simulink model "invertedPendolum"  (R2019b)
settings: Solver=VariableStepAuto  StartTime=0.0  StopTime=60  FixedStep=0.0001  RelTol=1e-4
InitFcn:
  | simulationVar
values from neighbouring files (symbols this model uses):
  tauMotMax = Ka * Id    (= 6208417600)    [simulationVar.m]
undefined symbols (not defined in the file or in its folder): smiData, X, Y, Z
libraries: sm_lib x768, simulink x6, nesl_utility x3
(part 1 of 13)
settings Model: Creator=alfyhack  LastModifiedBy=socci
settings SolverCC: AlgebraicLoopSolver=LineSearch
settings DebuggingCC: UnderSpecifiedDimensionMsg=warning
settings SFSimCC: CustomCodeUndefinedFunction=UseInterfaceOnly

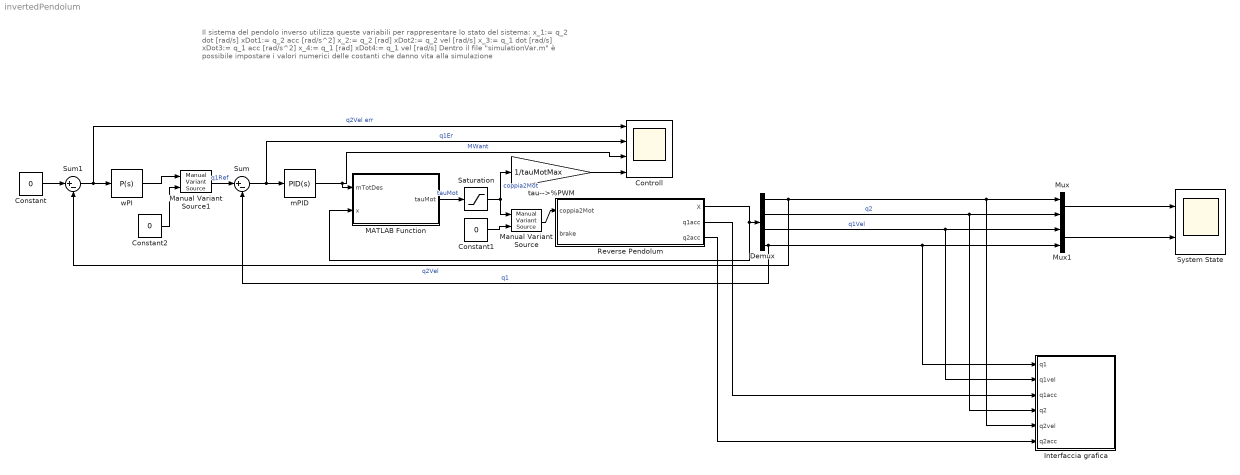
== system invertedPendolum ==
  note: Il sistema del pendolo inverso utilizza queste variabili per rappresentare lo stato del sistema:
      |
      | x_1:= q_2 dot  [rad/s]		xDot1:= q_2 acc   [rad/s^2]
      | x_2:= q_2        [rad]		xDot2:= q_2 vel    [rad/s]
      | x_3:= q_1 dot  [rad/s]		xDot3:= q_1 acc   [rad/s^2]
      | x_4:= q_1        [rad]		xDot4:= q_1 vel    [rad/s]
      |
      | Dentro il file "simulationVar.m" è possibile impostare i valori numerici delle costanti che danno vita alla simulazione
  Constant : Constant  Value=0
  Constant1 : Constant  Value=0
  Constant2 : Constant  Value=0
  Controll : Scope  NumInputPorts=4
  Demux : Demux
  Interfaccia grafica : Subsystem
  MATLAB Function : MATLAB Function  TreatAsAtomicUnit=on
  Manual Variant Source : simulink/Signal Routing/Manual Variant Source  NumChoices=2  LabelModeActiveChoice=V_1
      settings: SourceProductName=Simulink
  Manual Variant Source1 : simulink/Signal Routing/Manual Variant Source  NumChoices=2  LabelModeActiveChoice=V_1
      settings: SourceProductName=Simulink
  Mux : Mux  Inputs=2
  Mux1 : Mux  Inputs=2
  Reverse Pendolum : Subsystem
  Saturation : Saturate  UpperLimit=tauMotMax  LowerLimit=-tauMotMax
  Sum : Sum  Inputs=|+-
  Sum1 : Sum  Inputs=|+-
  System State : Scope  NumInputPorts=2
  mPID : simulink/Continuous/PID Controller  Controller=PID  Form=Parallel  TimeDomain=Continuous-time  SampleTime=-1  IntegratorMethod=Forward Euler  FilterMethod=Forward Euler  ControllerParametersSource=internal  P=44059890.2523914  I=6444277.98639226  D=74154463.3015082  UseFilter=on  N=34.9657186034109  TunerSelectOption=Transfer Function Based (PID Tuner App)  InitialConditionSource=internal  InitialConditionForIntegrator=0  InitialConditionForFilter=0  DifferentiatorICPrevScaledInput=0  ExternalReset=none  TrackingMode=off  Kt=1  LimitOutput=off  UpperSaturationLimit=1000  LowerSaturationLimit=1000  LinearizeAsGain=off  AntiWindupMode=none  Kb=1  POutMin=[]  POutMax=[]  IOutMin=[]  IOutMax=[]  DOutMin=[]  DOutMax=[]  NOutMin=[]  NOutMax=[]  SumOutMin=[]  SumOutMax=[]  SaturationOutMin=[]  SaturationOutMax=[]  PParamMin=[]  PParamMax=[]  IParamMin=[]  IParamMax=[]  DParamMin=[]  DParamMax=[]  NParamMin=[]  NParamMax=[]  KbParamMin=[]  KbParamMax=[]  KtParamMin=[]  KtParamMax=[]  KbOutMin=[]  KbOutMax=[]  KtOutMin=[]  KtOutMax=[]  IntegratorOutMin=[]  IntegratorOutMax=[]  FilterOutMin=[]  FilterOutMax=[]  SumI1OutMin=[]  SumI1OutMax=[]  SumI2OutMin=[]  SumI2OutMax=[]  SumI3OutMin=[]  SumI3OutMax=[]  SumI4OutMin=[]  SumI4OutMax=[]  SumDOutMin=[]  SumDOutMax=[]  DifferentiatorOutMin=[]  DifferentiatorOutMax=[]  FilterDiffOutCoefMin=[]  FilterDiffOutCoefMax=[]  ReciprocalOutMin=[]  ReciprocalOutMax=[]  SumDenOutMin=[]  SumDenOutMax=[]  SumNumOutMin=[]  SumNumOutMax=[]  DivideOutMin=[]  DivideOutMax=[]  IntegratorContinuousStateAttributes=''  IntegratorStateMustResolveToSignalObject=off  IntegratorRTWStateStorageClass=Auto  FilterContinuousStateAttributes=''  FilterStateMustResolveToSignalObject=off  FilterRTWStateStorageClass=Auto  ParallelPVariant=InternalParameters  IdealPVariant=Disabled  IVariant=InternalParameters  DVariant=InternalParameters  IntegratorVariant=Continuous  SatVariant=Disabled  AWVariant=Passthrough  PCopyVariant=Disabled  TRVariant=Disabled  FdbkBlocksVariant=Forward  IdealPFdbkVariant=Disabled  SatFdbkVariant=Disabled  DerivativeFilterVariant=ContFilter  NVariant=InternalParameters  NCopyVariant=Disabled  FilterICVariant=InternalICsFilter  IntegratorICVariant=InternalICs  ExternalResetVariant=Disabled  TRSumVariant=Passthrough  SumFdbkVariant=Disabled  SumVariant=Sum_PID
  tau-->%PWM : Gain  Gain=1/tauMotMax
  wPI : simulink/Continuous/PID Controller  Controller=P  Form=Parallel  TimeDomain=Continuous-time  SampleTime=-1  IntegratorMethod=Forward Euler  FilterMethod=Forward Euler  ControllerParametersSource=internal  P=0.000273498312206375  I=0.001  D=1  UseFilter=on  N=2000  TunerSelectOption=Transfer Function Based (PID Tuner App)  InitialConditionSource=internal  InitialConditionForIntegrator=0  InitialConditionForFilter=0  DifferentiatorICPrevScaledInput=0  ExternalReset=none  TrackingMode=off  Kt=1  LimitOutput=on  UpperSaturationLimit=0.1  LowerSaturationLimit=-0.1  LinearizeAsGain=off  AntiWindupMode=none  Kb=1  POutMin=[]  POutMax=[]  IOutMin=[]  IOutMax=[]  DOutMin=[]  DOutMax=[]  NOutMin=[]  NOutMax=[]  SumOutMin=[]  SumOutMax=[]  SaturationOutMin=[]  SaturationOutMax=[]  PParamMin=[]  PParamMax=[]  IParamMin=[]  IParamMax=[]  DParamMin=[]  DParamMax=[]  NParamMin=[]  NParamMax=[]  KbParamMin=[]  KbParamMax=[]  KtParamMin=[]  KtParamMax=[]  KbOutMin=[]  KbOutMax=[]  KtOutMin=[]  KtOutMax=[]  IntegratorOutMin=[]  IntegratorOutMax=[]  FilterOutMin=[]  FilterOutMax=[]  SumI1OutMin=[]  SumI1OutMax=[]  SumI2OutMin=[]  SumI2OutMax=[]  SumI3OutMin=[]  SumI3OutMax=[]  SumI4OutMin=[]  SumI4OutMax=[]  SumDOutMin=[]  SumDOutMax=[]  DifferentiatorOutMin=[]  DifferentiatorOutMax=[]  FilterDiffOutCoefMin=[]  FilterDiffOutCoefMax=[]  ReciprocalOutMin=[]  ReciprocalOutMax=[]  SumDenOutMin=[]  SumDenOutMax=[]  SumNumOutMin=[]  SumNumOutMax=[]  DivideOutMin=[]  DivideOutMax=[]  IntegratorContinuousStateAttributes=''  IntegratorStateMustResolveToSignalObject=off  IntegratorRTWStateStorageClass=Auto  FilterContinuousStateAttributes=''  FilterStateMustResolveToSignalObject=off  FilterRTWStateStorageClass=Auto  ParallelPVariant=InternalParameters  IdealPVariant=Disabled  IVariant=Disabled  DVariant=Disabled  IntegratorVariant=Disabled  SatVariant=Enabled  AWVariant=Disabled  PCopyVariant=Disabled  TRVariant=Disabled  FdbkBlocksVariant=Forward  IdealPFdbkVariant=Disabled  SatFdbkVariant=Disabled  DerivativeFilterVariant=Disabled  NVariant=Disabled  NCopyVariant=Disabled_SignalSpec  FilterICVariant=Disabled  IntegratorICVariant=Disabled  ExternalResetVariant=Disabled  TRSumVariant=Passthrough  SumFdbkVariant=Disabled  SumVariant=Passthrough_P
  wires:
  Demux/4 -> Interfaccia grafica/1(q1), Mux1/2, Sum/2  "q1"
  Demux/1 -> Interfaccia grafica/5(q2vel), Mux/1, Sum1/2  "q2Vel"
  MATLAB Function/1(tauMot) -> Saturation/1  "tauMot"
  mPID/1 -> Controll/3, MATLAB Function/1(mTotDes)  "MWant"
  Sum/1 -> Controll/2, mPID/1  "q1Er"
  wPI/1 -> Manual Variant Source1/1
  Constant/1 -> Sum1/1
  Sum1/1 -> Controll/1, wPI/1  "q2Vel err"
  Saturation/1 -> tau-->%PWM/1, Manual Variant Source/1  "coppia2Mot"
  Reverse Pendolum/1(X) -> Demux/1, MATLAB Function/2(x)
  Demux/3 -> Interfaccia grafica/2(q1vel), Mux1/1  "q1Vel"
  Mux1/1 -> System State/2
  Mux/1 -> System State/1
  tau-->%PWM/1 -> Controll/4
  Manual Variant Source/1 -> Reverse Pendolum/1(coppia2Mot)
  Constant1/1 -> Manual Variant Source/2
  Manual Variant Source1/1 -> Sum/1  "q1Ref"
  Constant2/1 -> Manual Variant Source1/2
  Demux/2 -> Interfaccia grafica/4(q2), Mux/2  "q2"
  Reverse Pendolum/2(q1acc) -> Interfaccia grafica/3(q1acc)
  Reverse Pendolum/3(q2acc) -> Interfaccia grafica/6(q2acc)

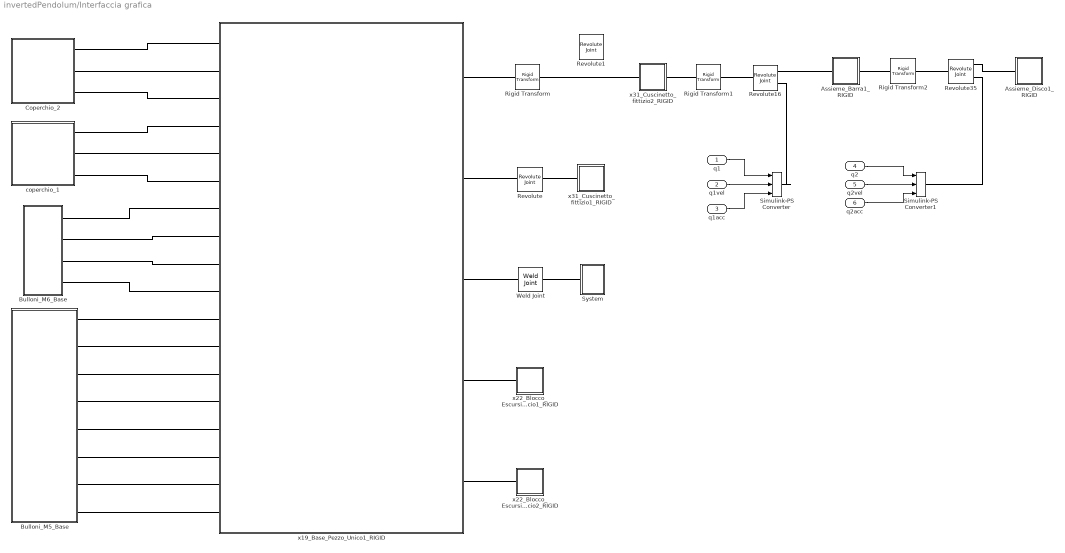
== system invertedPendolum/Interfaccia grafica ==
  q1 : Inport
  q1vel : Inport  Port=2
  q1acc : Inport  Port=3
  q2 : Inport  Port=4
  q2vel : Inport  Port=5
  q2acc : Inport  Port=6
  Assieme_Barra1_RIGID : Subsystem
  Assieme_Disco1_RIGID : Subsystem
  Bulloni_M5_Base : Subsystem
  Bulloni_M6_Base : Subsystem
  Coperchio_2 : Subsystem
  Revolute : sm_lib/Joints/Revolute Joint  JointMode=Normal  SenseConstraintForce=off  SenseConstraintForceX=off  SenseConstraintForceY=off  SenseConstraintForceZ=off  SenseConstraintTorque=off  SenseConstraintTorqueX=off  SenseConstraintTorqueY=off  SenseConstraintTorqueZ=off  SenseTotalForce=off  SenseTotalForceX=off  SenseTotalForceY=off  SenseTotalForceZ=off  SenseTotalTorque=off  SenseTotalTorqueX=off  SenseTotalTorqueY=off  SenseTotalTorqueZ=off  CompositeWrenchDir=FollowerOnBase  CompositeWrenchFrame=BaseFrame  EquilibriumPosition=0  EquilibriumPositionUnits=rad  SpringStiffness=0  SpringStiffnessUnits=N*m/rad  DampingCoefficient=0  DampingCoefficientUnits=N*m/(rad/s)  TorqueActuationMode=NoTorque  MotionActuationMode=ComputedMotion  SensePosition=off  SenseVelocity=off  SenseAcceleration=off  SenseTorqueForce=off  SenseLowerLimitTorqueForce=off  SenseUpperLimitTorqueForce=off  LowerLimitSpecify=off  LowerLimitBound=-90  LowerLimitBoundUnits=deg  LowerLimitStiffness=1e4  LowerLimitStiffnessUnits=N*m/deg  LowerLimitDamping=10  LowerLimitDampingUnits=N*m/(deg/s)  LowerLimitTransitionRegionWidth=0.1  LowerLimitTransitionRegionWidthUnits=deg  UpperLimitSpecify=off  UpperLimitBound=90  UpperLimitBoundUnits=deg  UpperLimitStiffness=1e4  UpperLimitStiffnessUnits=N*m/deg  UpperLimitDamping=10  UpperLimitDampingUnits=N*m/(deg/s)  UpperLimitTransitionRegionWidth=0.1  UpperLimitTransitionRegionWidthUnits=deg  PositionTargetSpecify=on  PositionTargetPriority=Low  PositionTargetValue=smiData.RevoluteJoint(1).Rz.Pos  PositionTargetValueUnits=deg  VelocityTargetSpecify=off  VelocityTargetPriority=High  VelocityTargetValue=0  VelocityTargetValueUnits=deg/s
  Revolute1 : sm_lib/Joints/Revolute Joint  JointMode=Normal  SenseConstraintForce=off  SenseConstraintForceX=off  SenseConstraintForceY=off  SenseConstraintForceZ=off  SenseConstraintTorque=off  SenseConstraintTorqueX=off  SenseConstraintTorqueY=off  SenseConstraintTorqueZ=off  SenseTotalForce=off  SenseTotalForceX=off  SenseTotalForceY=off  SenseTotalForceZ=off  SenseTotalTorque=off  SenseTotalTorqueX=off  SenseTotalTorqueY=off  SenseTotalTorqueZ=off  CompositeWrenchDir=FollowerOnBase  CompositeWrenchFrame=BaseFrame  EquilibriumPosition=0  EquilibriumPositionUnits=rad  SpringStiffness=0  SpringStiffnessUnits=N*m/rad  DampingCoefficient=0  DampingCoefficientUnits=N*m/(rad/s)  TorqueActuationMode=NoTorque  MotionActuationMode=ComputedMotion  SensePosition=off  SenseVelocity=off  SenseAcceleration=off  SenseTorqueForce=off  SenseLowerLimitTorqueForce=off  SenseUpperLimitTorqueForce=off  LowerLimitSpecify=off  LowerLimitBound=-90  LowerLimitBoundUnits=deg  LowerLimitStiffness=1e4  LowerLimitStiffnessUnits=N*m/deg  LowerLimitDamping=10  LowerLimitDampingUnits=N*m/(deg/s)  LowerLimitTransitionRegionWidth=0.1  LowerLimitTransitionRegionWidthUnits=deg  UpperLimitSpecify=off  UpperLimitBound=90  UpperLimitBoundUnits=deg  UpperLimitStiffness=1e4  UpperLimitStiffnessUnits=N*m/deg  UpperLimitDamping=10  UpperLimitDampingUnits=N*m/(deg/s)  UpperLimitTransitionRegionWidth=0.1  UpperLimitTransitionRegionWidthUnits=deg  PositionTargetSpecify=on  PositionTargetPriority=Low  PositionTargetValue=smiData.RevoluteJoint(2).Rz.Pos  PositionTargetValueUnits=deg  VelocityTargetSpecify=off  VelocityTargetPriority=High  VelocityTargetValue=0  VelocityTargetValueUnits=deg/s
  Revolute16 : sm_lib/Joints/Revolute Joint  JointMode=Normal  SenseConstraintForce=off  SenseConstraintForceX=off  SenseConstraintForceY=off  SenseConstraintForceZ=off  SenseConstraintTorque=off  SenseConstraintTorqueX=off  SenseConstraintTorqueY=off  SenseConstraintTorqueZ=off  SenseTotalForce=off  SenseTotalForceX=off  SenseTotalForceY=off  SenseTotalForceZ=off  SenseTotalTorque=off  SenseTotalTorqueX=off  SenseTotalTorqueY=off  SenseTotalTorqueZ=off  CompositeWrenchDir=FollowerOnBase  CompositeWrenchFrame=BaseFrame  EquilibriumPosition=0  EquilibriumPositionUnits=rad  SpringStiffness=0  SpringStiffnessUnits=N*m/rad  DampingCoefficient=0  DampingCoefficientUnits=N*m/(rad/s)  TorqueActuationMode=ComputedTorque  MotionActuationMode=InputMotion  SensePosition=off  SenseVelocity=off  SenseAcceleration=off  SenseTorqueForce=off  SenseLowerLimitTorqueForce=off  SenseUpperLimitTorqueForce=off  LowerLimitSpecify=off  LowerLimitBound=-90  LowerLimitBoundUnits=deg  LowerLimitStiffness=1e4  LowerLimitStiffnessUnits=N*m/deg  LowerLimitDamping=10  LowerLimitDampingUnits=N*m/(deg/s)  LowerLimitTransitionRegionWidth=0.1  LowerLimitTransitionRegionWidthUnits=deg  UpperLimitSpecify=off  UpperLimitBound=90  UpperLimitBoundUnits=deg  UpperLimitStiffness=1e4  UpperLimitStiffnessUnits=N*m/deg  UpperLimitDamping=10  UpperLimitDampingUnits=N*m/(deg/s)  UpperLimitTransitionRegionWidth=0.1  UpperLimitTransitionRegionWidthUnits=deg  PositionTargetSpecify=on  PositionTargetPriority=Low  PositionTargetValue=smiData.RevoluteJoint(17).Rz.Pos  PositionTargetValueUnits=deg  VelocityTargetSpecify=off  VelocityTargetPriority=High  VelocityTargetValue=0  VelocityTargetValueUnits=deg/s
  Revolute35 : sm_lib/Joints/Revolute Joint  JointMode=Normal  SenseConstraintForce=off  SenseConstraintForceX=off  SenseConstraintForceY=off  SenseConstraintForceZ=off  SenseConstraintTorque=off  SenseConstraintTorqueX=off  SenseConstraintTorqueY=off  SenseConstraintTorqueZ=off  SenseTotalForce=off  SenseTotalForceX=off  SenseTotalForceY=off  SenseTotalForceZ=off  SenseTotalTorque=off  SenseTotalTorqueX=off  SenseTotalTorqueY=off  SenseTotalTorqueZ=off  CompositeWrenchDir=FollowerOnBase  CompositeWrenchFrame=BaseFrame  EquilibriumPosition=0  EquilibriumPositionUnits=rad  SpringStiffness=0  SpringStiffnessUnits=N*m/rad  DampingCoefficient=0  DampingCoefficientUnits=N*m/(rad/s)  TorqueActuationMode=ComputedTorque  MotionActuationMode=InputMotion  SensePosition=off  SenseVelocity=off  SenseAcceleration=off  SenseTorqueForce=off  SenseLowerLimitTorqueForce=off  SenseUpperLimitTorqueForce=off  LowerLimitSpecify=off  LowerLimitBound=-90  LowerLimitBoundUnits=deg  LowerLimitStiffness=1e4  LowerLimitStiffnessUnits=N*m/deg  LowerLimitDamping=10  LowerLimitDampingUnits=N*m/(deg/s)  LowerLimitTransitionRegionWidth=0.1  LowerLimitTransitionRegionWidthUnits=deg  UpperLimitSpecify=off  UpperLimitBound=90  UpperLimitBoundUnits=deg  UpperLimitStiffness=1e4  UpperLimitStiffnessUnits=N*m/deg  UpperLimitDamping=10  UpperLimitDampingUnits=N*m/(deg/s)  UpperLimitTransitionRegionWidth=0.1  UpperLimitTransitionRegionWidthUnits=deg  PositionTargetSpecify=on  PositionTargetPriority=Low  PositionTargetValue=smiData.RevoluteJoint(36).Rz.Pos  PositionTargetValueUnits=deg  VelocityTargetSpecify=off  VelocityTargetPriority=High  VelocityTargetValue=0  VelocityTargetValueUnits=deg/s
  Rigid Transform : sm_lib/Frames and Transforms/Rigid Transform  TranslationMethod=None  TranslationStandardOffset=0  TranslationLengthUnit=m  TranslationStandardAxis=+Z  TranslationCartesianOffset=[0 0 0]  TranslationROffset=0  TranslationROffsetUnits=m  TranslationZOffset=0  TranslationZOffsetUnits=m  TranslationThetaOffset=0  TranslationThetaOffsetUnits=deg  RotationMethod=None  RotationAngleUnits=deg  RotationStandardAxis=+Z  RotationAngle=0.0  RotationArbitraryAxis=[0 0 1]  FollAlignAxisA=+X  BaseAlignAxisA=+Y  FollAlignAxisB=+Y  BaseAlignAxisB=+Z  RotationSequenceAxes=FollowerAxes  RotationSequence=XYX  RotationSequenceAngles=[0 0 0]  RotationSequenceAnglesUnits=deg  RotationMatrix=[1 0 0; 0 1 0; 0 0 1]
  Rigid Transform1 : sm_lib/Frames and Transforms/Rigid Transform  TranslationMethod=None  TranslationStandardOffset=0  TranslationLengthUnit=m  TranslationStandardAxis=+Z  TranslationCartesianOffset=[0 0 0]  TranslationROffset=0  TranslationROffsetUnits=m  TranslationZOffset=0  TranslationZOffsetUnits=m  TranslationThetaOffset=0  TranslationThetaOffsetUnits=deg  RotationMethod=None  RotationAngleUnits=deg  RotationStandardAxis=+Z  RotationAngle=0.0  RotationArbitraryAxis=[0 0 1]  FollAlignAxisA=+X  BaseAlignAxisA=+Y  FollAlignAxisB=+Y  BaseAlignAxisB=+Z  RotationSequenceAxes=FollowerAxes  RotationSequence=XYX  RotationSequenceAngles=[0 0 0]  RotationSequenceAnglesUnits=deg  RotationMatrix=[1 0 0; 0 1 0; 0 0 1]
  Rigid Transform2 : sm_lib/Frames and Transforms/Rigid Transform  TranslationMethod=None  TranslationStandardOffset=0  TranslationLengthUnit=m  TranslationStandardAxis=+Z  TranslationCartesianOffset=[0 0 0]  TranslationROffset=0  TranslationROffsetUnits=m  TranslationZOffset=0  TranslationZOffsetUnits=m  TranslationThetaOffset=0  TranslationThetaOffsetUnits=deg  RotationMethod=None  RotationAngleUnits=deg  RotationStandardAxis=+Z  RotationAngle=0.0  RotationArbitraryAxis=[0 0 1]  FollAlignAxisA=+X  BaseAlignAxisA=+Y  FollAlignAxisB=+Y  BaseAlignAxisB=+Z  RotationSequenceAxes=FollowerAxes  RotationSequence=XYX  RotationSequenceAngles=[0 0 0]  RotationSequenceAnglesUnits=deg  RotationMatrix=[1 0 0; 0 1 0; 0 0 1]
  Simulink-PS Converter : nesl_utility/Simulink-PS Converter  PhysicalDomain=network_engine_domain  SubClassName=ps_input  LeftPortType=input  RightPortType=output  PseudoPeriodic=off  Frequencies=[]  NoiseDistribution=none  NoiseParameters=[]  Unit=1  AffineConversion=off  FilteringAndDerivatives=provide  SimscapeFilterOrder=1  InputFilterTimeConstant=0.001  UdotUserProvided=2
  Simulink-PS Converter1 : nesl_utility/Simulink-PS Converter  PhysicalDomain=network_engine_domain  SubClassName=ps_input  LeftPortType=input  RightPortType=output  PseudoPeriodic=off  Frequencies=[]  NoiseDistribution=none  NoiseParameters=[]  Unit=1  AffineConversion=off  FilteringAndDerivatives=provide  SimscapeFilterOrder=1  InputFilterTimeConstant=0.001  UdotUserProvided=2
  System : Subsystem
  Weld Joint : sm_lib/Joints/Weld Joint  JointMode=Normal  SenseConstraintForce=off  SenseConstraintForceX=off  SenseConstraintForceY=off  SenseConstraintForceZ=off  SenseConstraintTorque=off  SenseConstraintTorqueX=off  SenseConstraintTorqueY=off  SenseConstraintTorqueZ=off  SenseTotalForce=off  SenseTotalForceX=off  SenseTotalForceY=off  SenseTotalForceZ=off  SenseTotalTorque=off  SenseTotalTorqueX=off  SenseTotalTorqueY=off  SenseTotalTorqueZ=off  CompositeWrenchDir=FollowerOnBase  CompositeWrenchFrame=BaseFrame
  coperchio_1 : Subsystem
  x19_Base_Pezzo_Unico1_RIGID : Subsystem
  x22_Blocco_Escursione_Braccio1_RIGID : Subsystem
  x22_Blocco_Escursione_Braccio2_RIGID : Subsystem
  x31_Cuscinetto_fittizio1_RIGID : Subsystem
  x31_Cuscinetto_fittizio2_RIGID : Subsystem
  wires:
  q1/1 -> Simulink-PS Converter/1
  q1vel/1 -> Simulink-PS Converter/2
  q1acc/1 -> Simulink-PS Converter/3
  q2/1 -> Simulink-PS Converter1/1
  q2vel/1 -> Simulink-PS Converter1/2
  q2acc/1 -> Simulink-PS Converter1/3
  connections:
  Bulloni_M5_Base/RConn4 -- x19_Base_Pezzo_Unico1_RIGID/LConn14
  Bulloni_M5_Base/RConn2 -- x19_Base_Pezzo_Unico1_RIGID/LConn12
  Bulloni_M6_Base/RConn1 -- x19_Base_Pezzo_Unico1_RIGID/LConn7
  coperchio_1/LConn1 -- x19_Base_Pezzo_Unico1_RIGID/LConn4
  Bulloni_M5_Base/RConn1 -- x19_Base_Pezzo_Unico1_RIGID/LConn11
  Coperchio_2/RConn2 -- x19_Base_Pezzo_Unico1_RIGID/LConn2
  Bulloni_M5_Base/RConn5 -- x19_Base_Pezzo_Unico1_RIGID/LConn15
  Bulloni_M5_Base/RConn6 -- x19_Base_Pezzo_Unico1_RIGID/LConn16
  Bulloni_M5_Base/RConn7 -- x19_Base_Pezzo_Unico1_RIGID/LConn17
  x22_Blocco_Escursione_Braccio1_RIGID/LConn1 -- x19_Base_Pezzo_Unico1_RIGID/RConn4
  Revolute/RConn1 -- x19_Base_Pezzo_Unico1_RIGID/RConn2
  coperchio_1/LConn3 -- x19_Base_Pezzo_Unico1_RIGID/LConn6
  Bulloni_M6_Base/RConn2 -- x19_Base_Pezzo_Unico1_RIGID/LConn8
  Weld Joint/LConn1 -- x19_Base_Pezzo_Unico1_RIGID/RConn3
  Bulloni_M5_Base/RConn3 -- x19_Base_Pezzo_Unico1_RIGID/LConn13
  Assieme_Disco1_RIGID/RConn1 -- Revolute35/LConn1
  Bulloni_M6_Base/RConn3 -- x19_Base_Pezzo_Unico1_RIGID/LConn9
  x19_Base_Pezzo_Unico1_RIGID/LConn18 -- Bulloni_M5_Base/RConn8
  coperchio_1/LConn2 -- x19_Base_Pezzo_Unico1_RIGID/LConn5
  Assieme_Barra1_RIGID/RConn1 -- Revolute16/LConn1
  x22_Blocco_Escursione_Braccio2_RIGID/LConn1 -- x19_Base_Pezzo_Unico1_RIGID/RConn5
  Bulloni_M6_Base/RConn4 -- x19_Base_Pezzo_Unico1_RIGID/LConn10
  Rigid Transform/LConn1 -- x19_Base_Pezzo_Unico1_RIGID/RConn1
  Revolute/LConn1 -- x31_Cuscinetto_fittizio1_RIGID/RConn1
  Coperchio_2/RConn1 -- x19_Base_Pezzo_Unico1_RIGID/LConn1
  Assieme_Barra1_RIGID/LConn1 -- Rigid Transform2/LConn1
  System/RConn1 -- Weld Joint/RConn1
  Rigid Transform1/LConn1 -- x31_Cuscinetto_fittizio2_RIGID/LConn1
  x19_Base_Pezzo_Unico1_RIGID/LConn3 -- Coperchio_2/RConn3
  Revolute16/RConn1 -- Rigid Transform1/RConn1
  Simulink-PS Converter/RConn1 -- Revolute16/LConn2
  Rigid Transform/RConn1 -- x31_Cuscinetto_fittizio2_RIGID/RConn1
  Simulink-PS Converter1/RConn1 -- Revolute35/LConn2
  Rigid Transform2/RConn1 -- Revolute35/RConn1

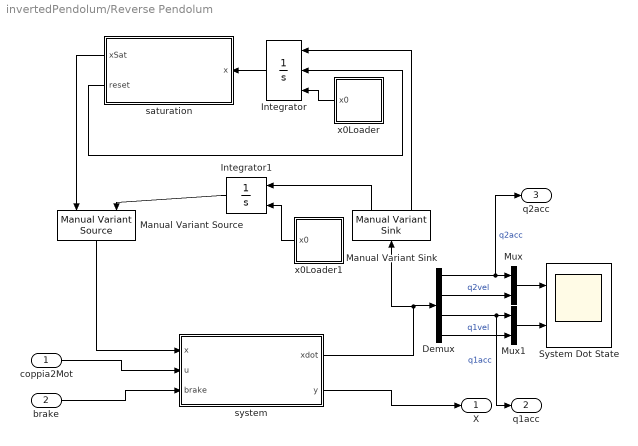
== system invertedPendolum/Reverse Pendolum ==
  coppia2Mot : Inport
  brake : Inport  Port=2
  Demux : Demux
  Integrator : Integrator  ExternalReset=rising  InitialConditionSource=external  InitialCondition=[0,0.1,0]
  Integrator1 : Integrator  InitialConditionSource=external
  Manual Variant Sink : simulink/Signal Routing/Manual Variant Sink  NumChoices=2  LabelModeActiveChoice=V_2
      settings: SourceProductName=Simulink
  Manual Variant Source : simulink/Signal Routing/Manual Variant Source  NumChoices=2  LabelModeActiveChoice=V_1
      settings: SourceProductName=Simulink
  Mux : Mux  Inputs=2
  Mux1 : Mux  Inputs=2
  System Dot State : Scope  NumInputPorts=2
  saturation : MATLAB Function  TreatAsAtomicUnit=on
  system : MATLAB Function  TreatAsAtomicUnit=on
  x0Loader : MATLAB Function  TreatAsAtomicUnit=on
  x0Loader1 : MATLAB Function  TreatAsAtomicUnit=on
  X : Outport  VectorParamsAs1DForOutWhenUnconnected=off
  q1acc : Outport  Port=2  VectorParamsAs1DForOutWhenUnconnected=off
  q2acc : Outport  Port=3  VectorParamsAs1DForOutWhenUnconnected=off
  wires:
  x0Loader/1(x0) -> Integrator/3
  Integrator/1 -> saturation/1(x)
  saturation/2(reset) -> Integrator/2
  coppia2Mot/1 -> system/2(u)
  system/2(y) -> X/1
  Mux/1 -> System Dot State/1
  Demux/3 -> q1acc/1, Mux1/1  "q1acc"
  Demux/1 -> q2acc/1, Mux/1  "q2acc"
  system/1(xdot) -> Manual Variant Sink/1, Demux/1
  Demux/2 -> Mux/2  "q2vel"
  Demux/4 -> Mux1/2  "q1vel"
  Mux1/1 -> System Dot State/2
  Manual Variant Sink/2 -> Integrator/1
  saturation/1(xSat) -> Manual Variant Source/1
  Integrator1/1 -> Manual Variant Source/2
  Manual Variant Sink/1 -> Integrator1/1
  Manual Variant Source/1 -> system/1(x)
  x0Loader1/1(x0) -> Integrator1/2
  brake/1 -> system/3(brake)
